simulink model "sampleModel1571"  (R2023a)
settings: Solver=VariableStepAuto  StartTime=0.0  StopTime=10.0  RelTol=1e-3
libraries: hdlsllib x9, simulink x2
settings Model: Creator=user1  LastModifiedBy=user1

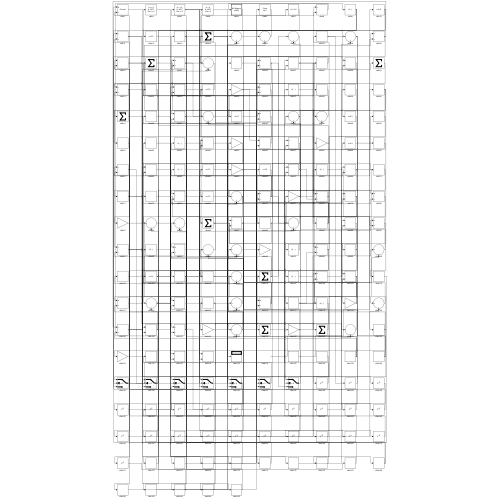
[thumbnail: Simulink's stored preview of the top-level diagram]
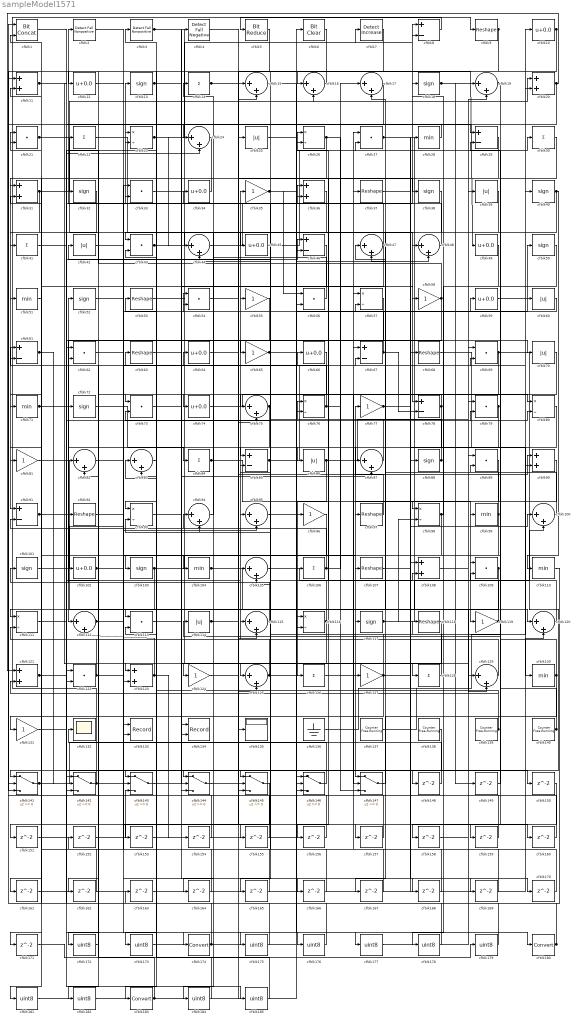
== system sampleModel1571 ==
  cfblk1 : hdlsllib/Logic and Bit Operations/Bit Concat  numInputs=2
  cfblk{10,12,34,45,49,59,64,66,74,102} (10 alike) : Bias  Bias=0.0  SaturateOnIntegerOverflow=off
  cfblk{15..17,19,24,44,47..48,75,82..83,87,94..95,100,105,112,115,120,125,129} (21 alike) : Sum  Inputs=|++
  cfblk{13,18,32,38,40,50,52,72,88,101,103,117} (12 alike) : Signum
  cfblk{28,51,71,99,104,110,130} (7 alike) : MinMax
  cfblk{14,22,30,41,84,106,126,128} (8 alike) : Sum  Inputs=+
  cfblk{9,37,53,63,68,92,97,107,118} (9 alike) : Reshape
  cfblk{11,20,31,36,90,108,121,123} (8 alike) : Sum
  cfblk{21,27,33,43,54,56,62,69,73,79,89,109,113,122} (14 alike) : DotProduct  OutDataTypeStr=Inherit: Inherit via internal rule
  cfblk{23,26,57,76,80,93,98,111,116} (9 alike) : Product  Inputs=*/  RndMeth=Zero  SaturateOnIntegerOverflow=on
  cfblk{25,39,42,60,70,86,114} (7 alike) : Abs  SaturateOnIntegerOverflow=off
  cfblk{35,55,58,65,77,81,96,119,124,127,131} (11 alike) : Gain
  cfblk132 : Scope
  cfblk133 : Record  FileSettingsInternal="{\"entries\":[{\"content\":{\"excelSettings\":{\"content\":{},\"type\":\"Streamout.ExcelSettings\"}},\"type\":\"Streamout.FileSettingStorage\",\"uuid\":\"\"}],\"packageUris\":[\"http:\\/\\/schema.mathworks.com\\/mf0\\/streamout_blocks\\/R2020a\"],\"version\":\"1.0\"}"  Layout=[1 1]  SignalsInternal="{\"entries\":[{\"content\":{\"signals\":[{\"content\":{\"blockPath\":[],\"dimensions\":[1],\"domain\":\"\",\"lineColor\":\"#a2142f\",\"plots\":[1],\"port\":1,\"signalID\":1850,\"signalName\":\"XY Graph:1\"},\"type\":\"RecordBlkView.Signal\",\"uuid\":\"\"},{\"content\":{\"blockPath\":[],\"dimensions\":[1],\"domain\":\"\",\"lineColor\":\"#139fff\",\"plots\":[1],\"port\":2,\"signalID\":1853,\"signalName\":\"XY Graph:2\"},\"type\":\"RecordBlkView.Signal\",\"uuid\":\"\"}]},\"type\":\"RecordBlkView.InputSignals\",\"uuid\":\"\"}],\"packageUris\":[\"http:\\/\\/schema.mathworks.com\\/mf0\\/streamout_blocks\\/R2020a\"],\"version\":\"1.0\"}"  VisualizationBindings="{\"xyplotplugin\":{\"info\":[{\"series\":[{\"bindingParametersList\":[{\"parameter\":\"X-Axis\",\"signalID\":1850,\"signalName\":\"XY Graph:1\"},{\"parameter\":\"Y-Axis\",\"signalID\":1853,\"signalName\":\"XY Graph:2\"}],\"seriesID\":15361}],\"subplotID\":1}]}}"  CompatibilityTag=XY  st=-1
  cfblk134 : Record  FileSettingsInternal="{\"entries\":[{\"content\":{\"excelSettings\":{\"content\":{},\"type\":\"Streamout.ExcelSettings\"}},\"type\":\"Streamout.FileSettingStorage\",\"uuid\":\"\"}],\"packageUris\":[\"http:\\/\\/schema.mathworks.com\\/mf0\\/streamout_blocks\\/R2020a\"],\"version\":\"1.0\"}"  Layout=[1 1]  SignalsInternal="{\"entries\":[{\"content\":{\"signals\":[{\"content\":{\"blockPath\":[],\"dimensions\":[1],\"domain\":\"\",\"lineColor\":\"#a2142f\",\"plots\":[1],\"port\":1,\"signalID\":1858,\"signalName\":\"XY Graph:1\"},\"type\":\"RecordBlkView.Signal\",\"uuid\":\"\"},{\"content\":{\"blockPath\":[],\"dimensions\":[1],\"domain\":\"\",\"lineColor\":\"#139fff\",\"plots\":[1],\"port\":2,\"signalID\":1861,\"signalName\":\"XY Graph:2\"},\"type\":\"RecordBlkView.Signal\",\"uuid\":\"\"}]},\"type\":\"RecordBlkView.InputSignals\",\"uuid\":\"\"}],\"packageUris\":[\"http:\\/\\/schema.mathworks.com\\/mf0\\/streamout_blocks\\/R2020a\"],\"version\":\"1.0\"}"  VisualizationBindings="{\"xyplotplugin\":{\"info\":[{\"series\":[{\"bindingParametersList\":[{\"parameter\":\"X-Axis\",\"signalID\":1858,\"signalName\":\"XY Graph:1\"},{\"parameter\":\"Y-Axis\",\"signalID\":1861,\"signalName\":\"XY Graph:2\"}],\"seriesID\":19335}],\"subplotID\":1}]}}"  CompatibilityTag=XY  st=-1
  cfblk135 : Display
  cfblk136 : Ground
  cfblk{137..140} (4 alike) : hdlsllib/Sources/Counter Free-Running  NumBits=16  tsamp=-1
  cfblk{141..147} (7 alike) : Switch  SaturateOnIntegerOverflow=off  InputSameDT=off
  cfblk{148..171} (24 alike) : Delay  SampleTime=1
  cfblk{172..173,175..179,181..182,184..185} (11 alike) : DataTypeConversion  OutDataTypeStr=uint8  SaturateOnIntegerOverflow=off  RndMeth=Floor
  cfblk174 : DataTypeConversion  SaturateOnIntegerOverflow=off  RndMeth=Floor
  cfblk180 : DataTypeConversion  SaturateOnIntegerOverflow=off  RndMeth=Floor
  cfblk183 : DataTypeConversion  SaturateOnIntegerOverflow=off  RndMeth=Floor
  cfblk2 : hdlsllib/Logic and Bit Operations/Detect Fall Nonpositive  vinit=0  OutDataTypeStr=boolean
  cfblk{8,29,46,61,67,78,85,91} (8 alike) : Sum  Inputs=+-
  cfblk3 : hdlsllib/Logic and Bit Operations/Detect Fall Nonpositive  vinit=0  OutDataTypeStr=boolean
  cfblk4 : hdlsllib/Logic and Bit Operations/Detect Fall Negative  vinit=0  OutDataTypeStr=boolean
  cfblk5 : hdlsllib/Logic and Bit Operations/Bit Reduce  mode=AND
  cfblk6 : simulink/Logic and Bit Operations/Bit Clear  iBit=0
      settings: LibrarySourceBlock=|
      | hdlsllib/Logic and Bit
      | Operations/Bit Clear
  cfblk7 : simulink/Logic and Bit Operations/Detect Increase  vinit=0.0  OutDataTypeStr=boolean
      settings: LibrarySourceBlock=|
      | hdlsllib/Logic and Bit
      | Operations/Detect
      | Increase
  wires:
  cfblk130/1 -> cfblk109/2, cfblk167/1
  cfblk129/1 -> cfblk35/1
  cfblk89/1 -> cfblk119/1
  cfblk115/1 -> cfblk52/1
  cfblk69/1 -> cfblk143/1, cfblk147/2, cfblk29/2
  cfblk11/1 -> cfblk123/1, cfblk29/1
  cfblk47/1 -> cfblk2/1, cfblk65/1
  cfblk45/1 -> cfblk30/1
  cfblk58/1 -> cfblk112/1, cfblk22/1
  cfblk142/1 -> cfblk9/1, cfblk46/1
  cfblk76/1 -> cfblk66/1, cfblk14/1, cfblk87/1
  cfblk62/1 -> cfblk174/1
  cfblk32/1 -> cfblk91/1
  cfblk86/1 -> cfblk126/1, cfblk39/1
  cfblk87/1 -> cfblk42/1
  cfblk31/1 -> cfblk51/1, cfblk20/1
  cfblk25/1 -> cfblk96/1
  cfblk42/1 -> cfblk133/1
  cfblk111/1 -> cfblk36/1
  cfblk23/1 -> cfblk8/1, cfblk44/1
  cfblk18/1 -> cfblk49/1, cfblk149/1
  cfblk79/1 -> cfblk147/1, cfblk182/1
  cfblk74/1 -> cfblk80/1
  cfblk137/1 -> cfblk10/1
  cfblk27/1 -> cfblk120/1, cfblk90/2
  cfblk59/1 -> cfblk50/1
  cfblk66/1 -> cfblk75/1
  cfblk48/1 -> cfblk13/1
  cfblk65/1 -> cfblk7/1, cfblk168/1
  cfblk67/1 -> cfblk55/1, cfblk78/2
  cfblk3/1 -> cfblk128/1, cfblk129/2, cfblk58/1
  cfblk99/1 -> cfblk54/1, cfblk142/3
  cfblk7/1 -> cfblk43/1
  cfblk39/1 -> cfblk78/1
  cfblk116/1 -> cfblk94/1, cfblk144/2, cfblk93/2, cfblk85/2
  cfblk24/1 -> cfblk41/1
  cfblk44/1 -> cfblk8/2
  cfblk139/1 -> cfblk3/1, cfblk121/2, cfblk101/1
  cfblk102/1 -> cfblk133/2, cfblk104/1
  cfblk68/1 -> cfblk130/1
  cfblk22/1 -> cfblk88/1
  cfblk82/1 -> cfblk67/2
  cfblk55/1 -> cfblk113/1
  cfblk43/1 -> cfblk48/1, cfblk103/1
  cfblk81/1 -> cfblk129/1
  cfblk104/1 -> cfblk116/1, cfblk16/2
  cfblk40/1 -> cfblk97/1, cfblk110/1, cfblk164/1
  cfblk131/1 -> cfblk92/1
  cfblk50/1 -> cfblk98/1
  cfblk61/1 -> cfblk21/1, cfblk142/2
  cfblk17/1 -> cfblk125/1
  cfblk34/1 -> cfblk31/1
  cfblk71/1 -> cfblk79/2, cfblk185/1
  cfblk33/1 -> cfblk146/1
  cfblk83/1 -> cfblk183/1
  cfblk8/1 -> cfblk5/1
  cfblk35/1 -> cfblk27/2, cfblk56/1
  cfblk15/1 -> cfblk180/1
  cfblk85/1 -> cfblk40/1, cfblk165/1
  cfblk46/1 -> cfblk71/1
  cfblk95/1 -> cfblk60/1
  cfblk38/1 -> cfblk116/2
  cfblk120/1 -> cfblk61/1
  cfblk106/1 -> cfblk91/2, cfblk17/1
  cfblk78/1 -> cfblk74/1, cfblk85/1
  cfblk14/1 -> cfblk125/2, cfblk19/1, cfblk38/1
  cfblk144/1 -> cfblk25/1
  cfblk54/1 -> cfblk135/1
  cfblk52/1 -> cfblk95/2
  cfblk105/1 -> cfblk108/2
  cfblk98/1 -> cfblk18/1, cfblk122/2, cfblk145/3
  cfblk108/1 -> cfblk79/1
  cfblk51/1 -> cfblk111/1
  cfblk41/1 -> cfblk70/1
  cfblk119/1 -> cfblk26/1, cfblk44/2
  cfblk124/1 -> cfblk90/1
  cfblk107/1 -> cfblk68/1
  cfblk94/1 -> cfblk64/1
  cfblk140/1 -> cfblk114/1, cfblk118/1
  cfblk147/1 -> cfblk47/1
  cfblk128/1 -> cfblk94/2
  cfblk101/1 -> cfblk33/1
  cfblk30/1 -> cfblk123/2
  cfblk5/1 -> cfblk73/1
  cfblk16/1 -> cfblk12/1
  cfblk125/1 -> cfblk48/2, cfblk11/2
  cfblk77/1 -> cfblk28/1, cfblk17/2
  cfblk9/1 -> cfblk82/1, cfblk144/3, cfblk45/1
  cfblk100/1 -> cfblk59/1
  cfblk19/1 -> cfblk109/1, cfblk159/1
  cfblk91/1 -> cfblk124/1, cfblk146/2, cfblk24/2
  cfblk57/1 -> cfblk86/1
  cfblk109/1 -> cfblk131/1, cfblk158/1
  cfblk112/1 -> cfblk80/2, cfblk36/2, cfblk54/2
  cfblk13/1 -> cfblk134/1, cfblk153/1
  cfblk88/1 -> cfblk47/2, cfblk76/1, cfblk32/1
  cfblk141/1 -> cfblk37/1, cfblk46/2
  cfblk60/1 -> cfblk57/2
  cfblk146/1 -> cfblk102/1
  cfblk122/1 -> cfblk34/1, cfblk111/2
  cfblk97/1 -> cfblk77/1
  cfblk26/1 -> cfblk81/1, cfblk147/3
  cfblk126/1 -> cfblk127/1
  cfblk21/1 -> cfblk72/1, cfblk146/3
  cfblk36/1 -> cfblk93/1
  cfblk73/1 -> cfblk145/1
  cfblk84/1 -> cfblk99/1, cfblk106/1
  cfblk123/1 -> cfblk112/2, cfblk154/1
  cfblk90/1 -> cfblk117/1
  cfblk53/1 -> cfblk145/2
  cfblk93/1 -> cfblk134/2
  cfblk127/1 -> cfblk100/1, cfblk105/2, cfblk171/1
  cfblk75/1 -> cfblk73/2, cfblk173/1
  cfblk20/1 -> cfblk121/1, cfblk141/2
  cfblk28/1 -> cfblk24/1
  cfblk136/1 -> cfblk69/1
  cfblk103/1 -> cfblk107/1, cfblk87/2, cfblk181/1
  cfblk10/1 -> cfblk16/1, cfblk141/3
  cfblk117/1 -> cfblk100/2, cfblk98/2, cfblk20/2
  cfblk114/1 -> cfblk144/1, cfblk75/2
  cfblk113/1 -> cfblk69/2
  cfblk72/1 -> cfblk84/1
  cfblk121/1 -> cfblk23/1, cfblk105/1, cfblk150/1
  cfblk143/1 -> cfblk4/1
  cfblk56/1 -> cfblk33/2
  cfblk4/1 -> cfblk115/2
  cfblk138/1 -> cfblk141/1
  cfblk49/1 -> cfblk148/1
  cfblk148/1 -> cfblk27/1
  cfblk149/1 -> cfblk89/2
  cfblk145/1 -> cfblk151/1
  cfblk151/1 -> cfblk143/3
  cfblk153/1 -> cfblk26/2
  cfblk154/1 -> cfblk31/2
  cfblk80/1 -> cfblk155/1
  cfblk155/1 -> cfblk21/2
  cfblk29/1 -> cfblk156/1
  cfblk156/1 -> cfblk11/1
  cfblk92/1 -> cfblk157/1
  cfblk157/1 -> cfblk115/1
  cfblk158/1 -> cfblk19/2
  cfblk159/1 -> cfblk142/1
  cfblk64/1 -> cfblk160/1
  cfblk160/1 -> cfblk57/1
  cfblk96/1 -> cfblk161/1
  cfblk161/1 -> cfblk108/1
  cfblk70/1 -> cfblk162/1
  cfblk162/1 -> cfblk122/1
  cfblk110/1 -> cfblk163/1
  cfblk163/1 -> cfblk120/2
  cfblk164/1 -> cfblk113/2
  cfblk165/1 -> cfblk61/2
  cfblk63/1 -> cfblk166/1
  cfblk166/1 -> cfblk43/2
  cfblk167/1 -> cfblk67/1
  cfblk168/1 -> cfblk82/2
  cfblk37/1 -> cfblk169/1
  cfblk169/1 -> cfblk95/1
  cfblk12/1 -> cfblk170/1
  cfblk170/1 -> cfblk143/2
  cfblk6/1 -> cfblk172/1
  cfblk172/1 -> cfblk152/1
  cfblk173/1 -> cfblk6/1
  cfblk174/1 -> cfblk76/2, cfblk53/1
  cfblk2/1 -> cfblk175/1
  cfblk175/1 -> cfblk62/1
  cfblk152/1 -> cfblk176/1
  cfblk176/1 -> cfblk62/2
  cfblk1/1 -> cfblk177/1
  cfblk177/1 -> cfblk89/1
  cfblk150/1 -> cfblk178/1
  cfblk178/1 -> cfblk1/1
  cfblk171/1 -> cfblk179/1
  cfblk179/1 -> cfblk1/2
  cfblk180/1 -> cfblk23/2, cfblk63/1
  cfblk181/1 -> cfblk15/1
  cfblk182/1 -> cfblk15/2
  cfblk183/1 -> cfblk56/2, cfblk132/1
  cfblk118/1 -> cfblk184/1
  cfblk184/1 -> cfblk83/1
  cfblk185/1 -> cfblk83/2
